simulink subsystem "PD_nadir"  (R2021a)
settings: Solver=VariableStepAuto  StartTime=0.0  StopTime=10.0  RelTol=1e-3
undefined symbols (not defined in the file): alpha, beta, k3, Max_magmom, Min_magmom, n
libraries: sharedutil x3
settings Model: Creator=Laura  LastModifiedBy=Laura

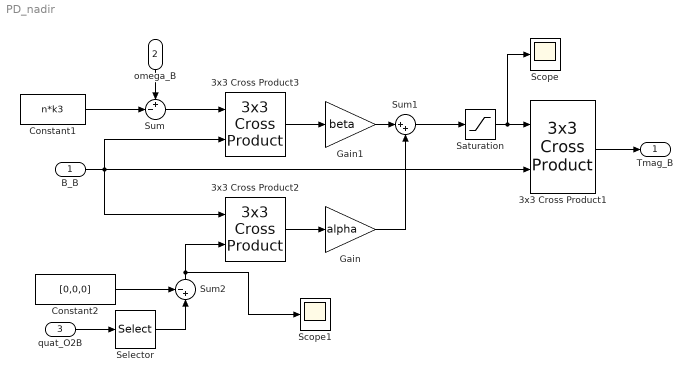
== system PD_nadir ==
  B_B : Inport
  omega_B : Inport  Port=2
  quat_O2B : Inport  Port=3
  3x3 Cross Product1 : sharedutil/3x3 Cross Product  aMode=aMode
      settings: SourceProductBaseCode=AE,PW,DR,MT,UV,VE
  3x3 Cross Product2 : sharedutil/3x3 Cross Product  aMode=aMode
      settings: SourceProductBaseCode=AE,PW,DR,MT,UV,VE
  3x3 Cross Product3 : sharedutil/3x3 Cross Product  aMode=aMode
      settings: SourceProductBaseCode=AE,PW,DR,MT,UV,VE
  Constant1 : Constant  Value=n*k3
  Constant2 : Constant  Value=[0,0,0]
  Gain : Gain  Gain=alpha
  Gain1 : Gain  Gain=beta
  Saturation : Saturate  UpperLimit=Max_magmom  LowerLimit=Min_magmom
  Scope : Scope
  Scope1 : Scope
  Selector : Selector  InputPortWidth=4  IndexOptions=Index vector (dialog)  Indices=[2 3 4]  OutputSizes=1
  Sum : Sum  Inputs=+-|
  Sum1 : Sum  Inputs=|++
  Sum2 : Sum  Inputs=-+|
  Tmag_B : Outport
  wires:
  3x3 Cross Product1/1 -> Tmag_B/1
  B_B/1 -> 3x3 Cross Product2/1, 3x3 Cross Product3/2, 3x3 Cross Product1/2
  quat_O2B/1 -> Selector/1
  3x3 Cross Product2/1 -> Gain/1
  3x3 Cross Product3/1 -> Gain1/1
  Saturation/1 -> Scope/1, 3x3 Cross Product1/1
  Constant1/1 -> Sum/2
  omega_B/1 -> Sum/1
  Sum/1 -> 3x3 Cross Product3/1
  Sum2/1 -> Scope1/1, 3x3 Cross Product2/2
  Selector/1 -> Sum2/2
  Constant2/1 -> Sum2/1
  Gain1/1 -> Sum1/1
  Sum1/1 -> Saturation/1
  Gain/1 -> Sum1/2
